simulink library "dlbsBlockSigmoid"  (R2025b)
settings: Solver=VariableStepAuto  StartTime=0.0  StopTime=10.0  RelTol=1e-3
libraries: dlbsBlockExtractGradientGF x1, dlbsBlockInsertGradientGF x1
settings Model: Creator=lt6037  LastModifiedBy=lt6037

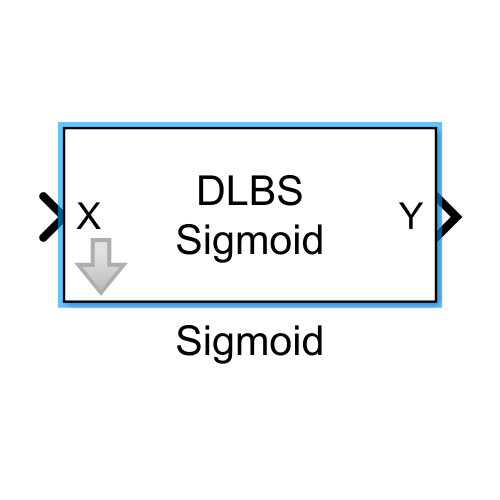
[thumbnail: Simulink's stored preview of the top-level diagram]
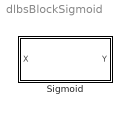
== system dlbsBlockSigmoid ==
  Sigmoid : Subsystem
      mask help: Applies the logistic sigmoid activation to the input tensor. The operation is applied element-wise across all tensor elements.
      mask Help: web("dlbsHelpBlockSigmoid.html")
      mask Display: fprintf("DLBS\nSigmoid")

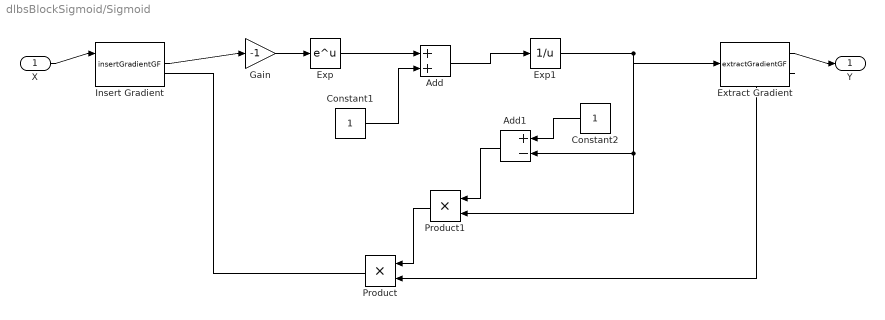
== system dlbsBlockSigmoid/Sigmoid ==
  X : Inport
  Add : Sum
  Add1 : Sum  Inputs=+-
  Constant1 : Constant
  Constant2 : Constant
  Exp : Math
  Exp1 : Math  Operator=reciprocal
  Extract Gradient : dlbsBlockExtractGradientGF/extractGradientGF
  Gain : Gain  Gain=-1
  Insert Gradient : dlbsBlockInsertGradientGF/insertGradientGF
  Product : Product
  Product1 : Product
  Y : Outport
  wires:
  Exp/1 -> Add/1
  Insert Gradient/1 -> Gain/1
  Exp1/1 -> Extract Gradient/1, Product1/2, Add1/2
  Add/1 -> Exp1/1
  Gain/1 -> Exp/1
  Product1/1 -> Product/1
  Add1/1 -> Product1/1
  Constant1/1 -> Add/2
  Constant2/1 -> Add1/1
  Product/1 -> Insert Gradient/2
  Extract Gradient/2 -> Product/2
  X/1 -> Insert Gradient/1
  Extract Gradient/1 -> Y/1
